simulink library "FilterLib"  (R2025a)
settings: Solver=VariableStepAuto  StartTime=0.0  StopTime=10.0  RelTol=1e-3
Description:
  | This block library contains common filters for use by models in the project.
settings Model: Creator=The MathWorks, Inc.  LastModifiedBy=The MathWorks, Inc.
settings SolverCC: AlgebraicLoopSolver=TrustRegion  MaxZcPerStep=1.0
settings DataIOCC: ReturnWorkspaceOutputs=off
settings DebuggingCC: UnconnectedInputMsg=warning  UnconnectedOutputMsg=warning  UnconnectedLineMsg=warning  PregeneratedLibrarySubsystemCodeDiagnostic=none  ArithmeticOperatorsInVariantConditions=warning
settings ModelReferenceCC: EnableRefExpFcnMdlSchedulingChecks=on
settings SFSimCC: SimUseLocalCustomCode=off  CustomCodeUndefinedFunction=UseInterfaceOnly
settings RTWCC: RTWUseLocalCustomCode=off  GPUComputeCapability=3.5  DLArmComputeVersion=19.05
settings CodeAppCC: StateflowObjectComments=on

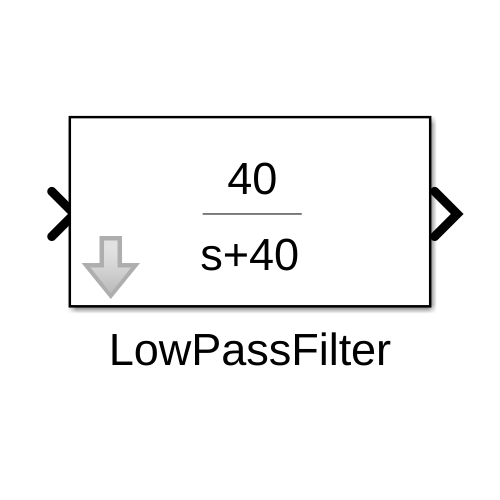
[thumbnail: Simulink's stored preview of the top-level diagram]
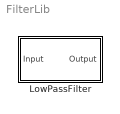
== system FilterLib ==
  LowPassFilter : Subsystem  mask(Low Pass Filter){fq=40, ts=0.01}
      mask prompts: fq "Roll-off frequency (rad/s)"; ts "Sample time"
      mask help: Discrete low pass filter
      mask init:
      | n2 = 0.329679953964361;
      | d2 = 0.670320046035639;
      | 
      | % num = fq;
      | % den = [1,fq];
      | % contSys = tf(num,den);
      | % if ts > 0
      | %     discSys = c2d(contSys,ts);
      | %     [n,d] = tfdata(discSys,'v');
      | %     n2 = n(2);
      | %     d2 = -d(2);
      | % else
      | %     error('Please specify a discrete sample time.');
      | % end
      mask Display: dpoly([0,fq],[1,fq]);

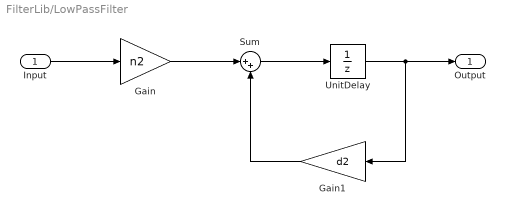
== system FilterLib/LowPassFilter ==
  Input : Inport
  Gain : Gain  Gain=n2
  Gain1 : Gain  Gain=d2
  Sum : Sum  Inputs=|++
  UnitDelay : UnitDelay  SampleTime=ts  HasFrameUpgradeWarning=on
  Output : Outport
  wires:
  Input/1 -> Gain/1
  Gain/1 -> Sum/1
  Sum/1 -> UnitDelay/1
  UnitDelay/1 -> Gain1/1, Output/1
  Gain1/1 -> Sum/2
